simulink model "WT_labor"  (R2023a)
settings: Solver=VariableStepAuto  StartTime=0.0  StopTime=inf  RelTol=1e-3
InitFcn:
  | WT_init
values from neighbouring files (symbols this model uses):
  a = A_out/A_t * sqrt((2*g)/(1+xi))    [WT_init.m]
  a1 = 3.744e-2    (= 0.03744)    [WT_init.m]
  a2 = 3.812e-2    (= 0.03812)    [WT_init.m]
  A_t = 50e-4    (= 0.005)    [WT_init.m]
  Gf_y = lambda^2/(s+lambda)^2    [WT_init.m]
  h2_rl = 5e-2    (= 0.05)    [WT_init.m]
  rho = 1000    [WT_init.m]
undefined symbols (not defined in the file or in its folder): National_Instruments, PCI, pid_tune_fast
libraries: sldrtlib x3, slpidlib x1
settings Model: Creator=marti  LastModifiedBy=EAL
settings RTWCC: GPUComputeCapability=5.0

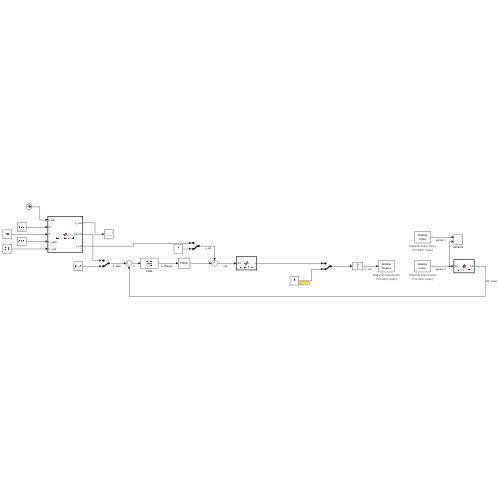
[thumbnail: Simulink's stored preview of the top-level diagram]
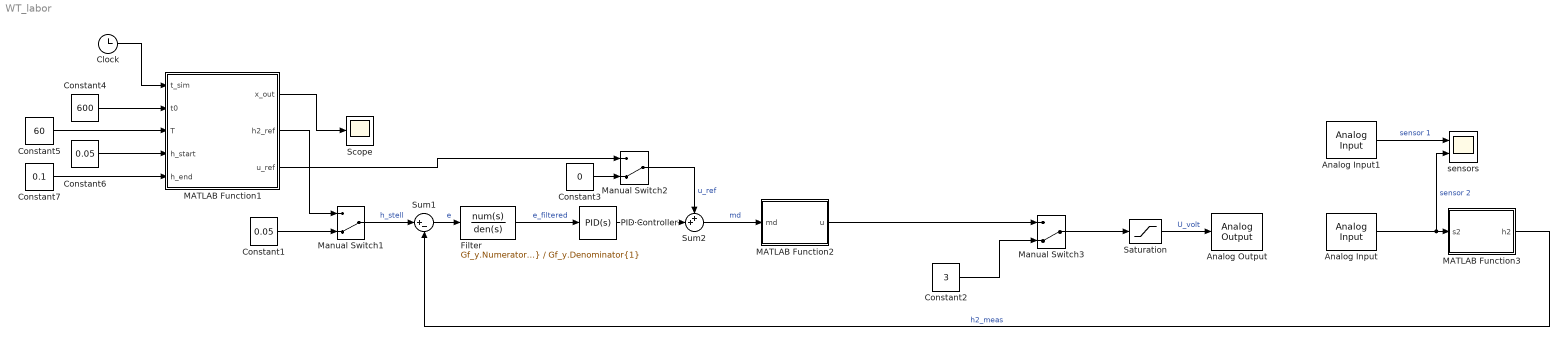
== system WT_labor ==
  Analog Input : sldrtlib/Analog Input  SampleTime=0.1  MaxMissedTicks=10  ShowMissedTicks=off  YieldWhenWaiting=off  DrvName=National_Instruments/PCI-6221  DrvAddress=4294967295  DrvOptions=[0 2 3 0 0]  Channels=2  RangeMode=1  VoltRange=1  DataType=1
      settings: AttributesFormatString=National Instruments\nPCI-6221 [auto]
  Analog Input1 : sldrtlib/Analog Input  SampleTime=0.1  MaxMissedTicks=10  ShowMissedTicks=off  YieldWhenWaiting=off  DrvName=National_Instruments/PCI-6221  DrvAddress=4294967295  DrvOptions=[0 2 3 0 0]  Channels=1  RangeMode=1  VoltRange=1  DataType=1
      settings: AttributesFormatString=National Instruments\nPCI-6221 [auto]
  Analog Output : sldrtlib/Analog Output  SampleTime=0.1  MaxMissedTicks=10  ShowMissedTicks=off  YieldWhenWaiting=off  DrvName=National_Instruments/PCI-6221  DrvAddress=4294967295  DrvOptions=[0 2 3 0 0]  Channels=2  RangeMode=1  VoltRange=1  InitialValue=[]  FinalValue=[]
      settings: AttributesFormatString=National Instruments\nPCI-6221 [auto]
  Clock : Clock
  Constant1 : Constant  Value=0.05
  Constant2 : Constant  Value=3
  Constant3 : Constant  Value=0
  Constant4 : Constant  Value=600
  Constant5 : Constant  Value=60
  Constant6 : Constant  Value=0.05
  Constant7 : Constant  Value=0.1
  Filter : TransferFcn  Numerator=Gf_y.Numerator{1}  Denominator=Gf_y.Denominator{1}
  MATLAB Function1 : MATLAB Function  TreatAsAtomicUnit=on
  MATLAB Function2 : MATLAB Function  TreatAsAtomicUnit=on
  MATLAB Function3 : MATLAB Function  TreatAsAtomicUnit=on
  Manual Switch1 : ManualSwitch  CurrentSetting=0
  Manual Switch2 : ManualSwitch  CurrentSetting=0
  Manual Switch3 : ManualSwitch  CurrentSetting=0
  PID Controller : slpidlib/PID Controller  Controller=PID  Form=Parallel  TimeDomain=Continuous-time  UseExternalTs=off  SampleTime=-1  IntegratorMethod=Forward Euler  FilterMethod=Forward Euler  ControllerParametersSource=internal  P=pid_tune_fast.Kp  I=pid_tune_fast.Ki  UseKiTs=off  D=pid_tune_fast.Kd  N=50  UseFilter=on  TunerSelectOption=Transfer Function Based (PID Tuner App)  InitialConditionSource=internal  InitialConditionForIntegrator=0  InitialConditionForFilter=0  DifferentiatorICPrevScaledInput=0  ExternalReset=none  TrackingMode=off  Kt=1  LimitOutput=off  SatLimitsSource=internal  UpperSaturationLimit=inf  LowerSaturationLimit=-inf  LinearizeAsGain=on  AntiWindupMode=none  Kb=1  LimitIntegrator=off  UpperIntegratorSaturationLimit=inf  LowerIntegratorSaturationLimit=-inf  POutMin=[]  POutMax=[]  IOutMin=[]  IOutMax=[]  DOutMin=[]  DOutMax=[]  NOutMin=[]  NOutMax=[]  SumOutMin=[]  SumOutMax=[]  SaturationOutMin=[]  SaturationOutMax=[]  PParamMin=[]  PParamMax=[]  IParamMin=[]  IParamMax=[]  DParamMin=[]  DParamMax=[]  NParamMin=[]  NParamMax=[]  KbParamMin=[]  KbParamMax=[]  KtParamMin=[]  KtParamMax=[]  KbOutMin=[]  KbOutMax=[]  KtOutMin=[]  KtOutMax=[]  IntegratorOutMin=[]  IntegratorOutMax=[]  FilterOutMin=[]  FilterOutMax=[]  SumI1OutMin=[]  SumI1OutMax=[]  SumI2OutMin=[]  SumI2OutMax=[]  SumI3OutMin=[]  SumI3OutMax=[]  SumI4OutMin=[]  SumI4OutMax=[]  SumDOutMin=[]  SumDOutMax=[]  DifferentiatorOutMin=[]  DifferentiatorOutMax=[]  FilterDiffOutCoefMin=[]  FilterDiffOutCoefMax=[]  ReciprocalOutMin=[]  ReciprocalOutMax=[]  SumDenOutMin=[]  SumDenOutMax=[]  SumNumOutMin=[]  SumNumOutMax=[]  DivideOutMin=[]  DivideOutMax=[]  UdiffTsProdOutMin=[]  UdiffTsProdOutMax=[]  NTsProdOutMin=[]  NTsProdOutMax=[]  UintegralTsProdOutMin=[]  UintegralTsProdOutMax=[]  UngainTsProdOutMin=[]  UngainTsProdOutMax=[]  ClampingZeroOutDataTypeStr=Inherit: Inherit via back propagation  ClampingZeroOutMin=[]  ClampingZeroOutMax=[]  FilterDenConstantOutDataTypeStr=Inherit: Inherit via back propagation  FilterDenConstantOutMin=[]  FilterDenConstantOutMax=[]  PCopyOutDataTypeStr=Inherit: Inherit via back propagation  PCopyOutMin=[]  PCopyOutMax=[]  NCopyOutDataTypeStr=Inherit: Inherit via back propagation  NCopyOutMin=[]  NCopyOutMax=[]  IntegratorContinuousStateAttributes=''  IntegratorStateMustResolveToSignalObject=off  IntegratorRTWStateStorageClass=Auto  FilterContinuousStateAttributes=''  FilterStateMustResolveToSignalObject=off  FilterRTWStateStorageClass=Auto  ParallelPVariant=InternalParameters  IdealPVariant=Disabled  IVariant=InternalParameters  DVariant=InternalParameters  IntegratorVariant=Continuous  SatVariant=Disabled  AWVariant=Passthrough  PCopyVariant=Disabled  TRVariant=Disabled  FdbkBlocksVariant=Forward  IdealPFdbkVariant=Disabled  SatFdbkVariant=Disabled  DerivativeFilterVariant=ContFilter  NVariant=InternalParameters  NCopyVariant=Disabled  FilterICVariant=InternalICsFilter  IntegratorICVariant=InternalICs  ExternalResetVariant=Disabled  TRSumVariant=Passthrough  SumFdbkVariant=Disabled  SumVariant=Sum_PID  TsampFilterVariant=InternalTs  TsampNgainVariant=Passthrough  TsampIntegralVariant=Disabled_SignalSpec  ExternalSaturationOutDataTypeStr=Inherit: Same as second input
  Saturation : Saturate  UpperLimit=5  LowerLimit=0
  Scope : Scope
  Sum1 : Sum  Inputs=|+-
  Sum2 : Sum  Inputs=++|
  sensors : Scope  NumInputPorts=2
  wires:
  Saturation/1 -> Analog Output/1  "U_volt"
  Constant1/1 -> Manual Switch1/2
  Sum1/1 -> Filter/1  "e"
  MATLAB Function3/1(h2) -> Sum1/2  "h2_meas"
  Sum2/1 -> MATLAB Function2/1(md)  "md"
  Clock/1 -> MATLAB Function1/1(t_sim)
  Manual Switch1/1 -> Sum1/1  "h_stell"
  MATLAB Function1/2(h2_ref) -> Manual Switch1/1
  MATLAB Function1/3(u_ref) -> Manual Switch2/1
  Manual Switch2/1 -> Sum2/1  "u_ref"
  MATLAB Function1/1(x_out) -> Scope/1
  PID Controller/1 -> Sum2/2
  Filter/1 -> PID Controller/1  "e_filtered"
  Analog Input/1 -> sensors/2, MATLAB Function3/1(s2)  "sensor 2"
  MATLAB Function2/1(u) -> Manual Switch3/1
  Constant2/1 -> Manual Switch3/2
  Manual Switch3/1 -> Saturation/1
  Constant3/1 -> Manual Switch2/2
  Constant4/1 -> MATLAB Function1/2(t0)
  Constant5/1 -> MATLAB Function1/3(T)
  Constant6/1 -> MATLAB Function1/4(h_start)
  Constant7/1 -> MATLAB Function1/5(h_end)
  Analog Input1/1 -> sensors/1  "sensor 1"

== matlab function WT_labor/MATLAB Function1 ==
  data: t_sim input; t0 input; T input; h_start input; h_end input; x_out output; h2_ref output; u_ref output; a parameter; rho parameter; A_t parameter; h2_rl parameter; a1 parameter; a2 parameter
function [x_out, h2_ref, u_ref] = feed_forward(t_sim, t0, T, h_start, h_end , a, rho, A_t, h2_rl, a1, a2)

% adjust time
t = t_sim-t0;

h2_0 = h_start; % initial height
h2_T = h_end; % target height

% functions
phi     = @(t) 35*t.^4 - 84*t.^5 + 70*t.^6 - 20*t.^7;
phi_d   = @(t) 140*t.^3 - 420*t.^4 + 420*t.^5 - 140*t.^6;
phi_dd  = @(t) 420*t.^2 - 1680*t.^3 + 2100*t.^4 - 840*t.^5;
% phi_ddd = @(t) 840*t - 5040*t.^2 + 8400*t.^3 - 4200*t.^4;

eta_d = 0;
eta_dd = 0;
% eta_ddd = 0;

if t<0
    eta = h2_0;
elseif t>T
    eta = h2_T;
else
    eta = h2_0 + (h2_T-h2_0) * phi(t/T);
    eta_d = (h2_T-h2_0) * phi_d(t/T)/T;
    eta_dd = (h2_T-h2_0) * phi_dd(t/T)/T^2;
    % eta_ddd = (h_T-h_0) * phi_ddd(t/T)/T^3;
end

% h1 = ((eta_d + a*sqrt(eta))/a)^2;
% h1_d = 2*((eta_d + a*sqrt(eta))/a)*1/a*eta_dd * ((eta_d + a*sqrt(eta))/a)*(1/sqrt(eta))*eta_d;
% u_ref = rho*A_t*(h1_d + a*sqrt(h1));


h1 = (eta_d + a2*sqrt(eta))^2 / a1^2;
h1_d = 2/a1^2 * (eta_d + a2*sqrt(eta)) * (eta_dd + a2*eta_d/(2*sqrt(eta)));
u_ref = rho*A_t * (h1_d + a1*sqrt(h1));

h2_ref = eta;

x_out = [h1; h2_ref];

== matlab function WT_labor/MATLAB Function2 ==
  data: md input; u output
function u = m_d_2_u(md)
k_pump = 0.0155;
u = md / k_pump;

== matlab function WT_labor/MATLAB Function3 ==
  data: s2 input; h2 output
function h2 = s2_2_h2(s2)
c = 0.1296;
b = -0.2793 + 0.005;
h2 = c * s2 + b;
